simulink model "fixFifoA"  (R2024b)
settings: Solver=VariableStepAuto  StartTime=0.0  StopTime=10.0  RelTol=1e-3
libraries: NSA_DEVS_LOGISTICS x5, NSA_DEVS_SINKS x4, NSA_DEVS_ROUTING x3, NSA_DEVS_MATH_OPERATIONS x1, NSA_DEVS_SOURCES x1
settings Model: Creator=david  LastModifiedBy=peter
settings OptimizationCC: ReuseModelBlockBuffer=off
settings RTWCC: GPUComputeCapability=3.5

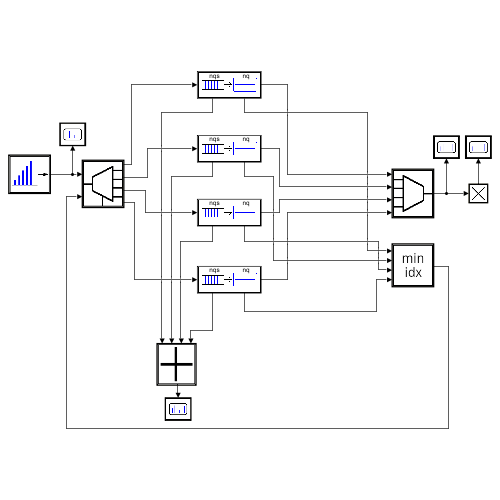
[thumbnail: Simulink's stored preview of the top-level diagram]
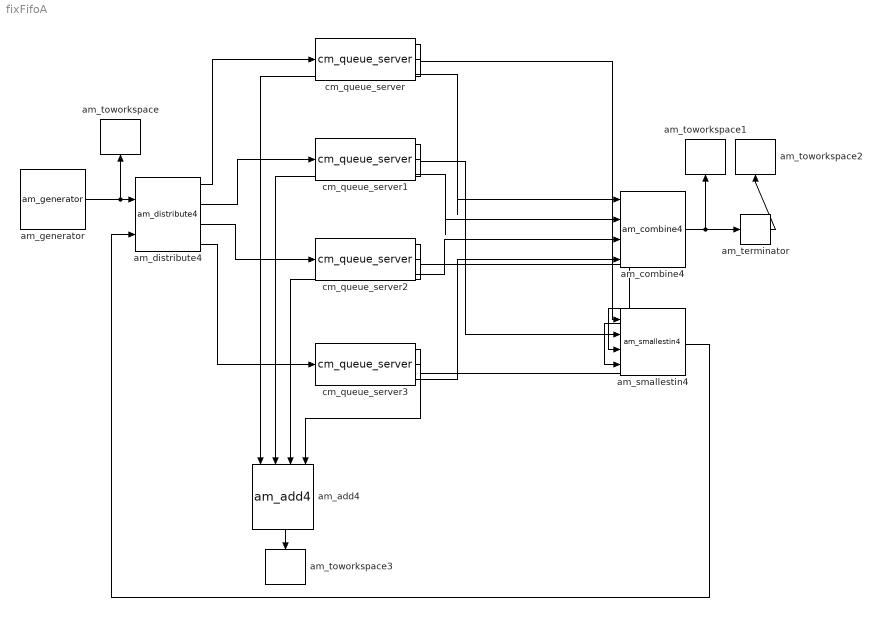
== system fixFifoA ==
  am_add4 : NSA_DEVS_MATH_OPERATIONS/am_add4  tau=[0,1]  debug=0
      settings: SourceProductName=Math Operations
  am_combine4 : NSA_DEVS_ROUTING/am_combine4  tD=[0,1]  tau=[0,1]  debug=0
      settings: SourceProductName=Routing
  am_distribute4 : NSA_DEVS_ROUTING/am_distribute4  port0=1  field="\"\""  tau=[0,3]  debug=0
      settings: SourceProductName=Routing
  am_generator : NSA_DEVS_SOURCES/am_generator  tG=1  n0=1  nG=100  tD=[0,2]  debug=0
      settings: SourceProductName=Sources
  am_smallestin4 : NSA_DEVS_ROUTING/am_smallestin4  val0=0  tau=[0,1]  debug=0
      settings: SourceProductName=Routing
  am_terminator : NSA_DEVS_LOGISTICS/am_terminator  tau=[0,1]  debug=0
      settings: SourceProductName=Logistics
  am_toworkspace : NSA_DEVS_SINKS/am_toworkspace  varname="\"gen_out\""  t0=0  format="\"vector\""  tau=[0,5]  debug=0
      settings: SourceProductName=Sinks
  am_toworkspace1 : NSA_DEVS_SINKS/am_toworkspace  varname="\"output\""  t0=0  format="\"vector\""  tau=[0,0.5]  debug=0
      settings: SourceProductName=Sinks
  am_toworkspace2 : NSA_DEVS_SINKS/am_toworkspace  varname="\"thrput\""  t0=0  format="\"vector\""  tau=[0,5]  debug=0
      settings: SourceProductName=Sinks
  am_toworkspace3 : NSA_DEVS_SINKS/am_toworkspace  varname="\"SUM_N\""  t0=0  format="\"vector\""  tau=[0,5]  debug=0
      settings: SourceProductName=Sinks
  cm_queue_server{,1..3} (4 alike) : NSA_DEVS_LOGISTICS/cm_queue_server  ts=4.5  tau=[0,1]  debug=0
      settings: SourceProductName=Logistics
  wires:
  am_generator/1 -> am_toworkspace/1, am_distribute4/1
  am_distribute4/1 -> cm_queue_server/1
  cm_queue_server/3 -> am_smallestin4/1
  cm_queue_server1/3 -> am_smallestin4/2
  cm_queue_server2/3 -> am_smallestin4/3
  cm_queue_server3/3 -> am_smallestin4/4
  am_smallestin4/1 -> am_distribute4/2
  cm_queue_server/1 -> am_combine4/1
  cm_queue_server2/1 -> am_combine4/3
  cm_queue_server3/1 -> am_combine4/4
  am_combine4/1 -> am_toworkspace1/1, am_terminator/1
  am_terminator/1 -> am_toworkspace2/1
  am_add4/1 -> am_toworkspace3/1
  cm_queue_server/2 -> am_add4/1
  cm_queue_server1/2 -> am_add4/2
  cm_queue_server2/2 -> am_add4/3
  cm_queue_server3/2 -> am_add4/4
  cm_queue_server1/1 -> am_combine4/2
  am_distribute4/2 -> cm_queue_server1/1
  am_distribute4/3 -> cm_queue_server2/1
  am_distribute4/4 -> cm_queue_server3/1
